simulink model "Smart_Grid_2"  (R2024b)
settings: Solver=FixedStepAuto  StartTime=0.0  StopTime=0.5  FixedStep=1e-5  RelTol=1e-3
undefined symbols (not defined in the file): Ion, Lithium
libraries: spsSeriesRLCBranchLib x76, spsRMSLib x65, spsIGBTDiodeLib x41, eeGeneralControl x36, slpidlib x34, spsThreePhaseVIMeasurementLib x32, spsVoltageMeasurementLib x18, simulink x16, spsCurrentMeasurementLib x15, spsThreePhaseBreakerLib x12, spsAlphaBetaZerotodq0Lib x12, spsPower3phPhasorLib x10
(part 3 of 8)

== system Smart_Grid_2/Battery_Farm, V2G 110KWH/Subsystem ==
  PWM1 : Inport
  PWM2 : Inport  Port=2
  PWM3 : Inport  Port=3
  PWM4 : Inport  Port=4
  PWM5 : Inport  Port=5
  PWM6 : Inport  Port=6
  IGBT/Diode{,1..5} (6 alike) : spsIGBTDiodeLib/IGBT//Diode  Ron=1e-3  Rs=1e5  Cs=inf  Measurements=off
  Series RLC Branch9 : spsSeriesRLCBranchLib/Series RLC Branch  LConnTagsString=__new0  RConnTagsString=__new0  BranchType=RC  Resistance=1e-3  Inductance=1e-3  SetiL0=off  InitialCurrent=0  Capacitance=5600e-6  Setx0=on  InitialVoltage=800  Measurements=None
  VR : PMIOPort  Side=Left
  VY : PMIOPort  Port=2  Side=Left
  VB : PMIOPort  Port=3  Side=Left
  VDC+ : PMIOPort  Port=4  Side=Right
  VDC- : PMIOPort  Port=5  Side=Right
  wires:
  PWM5/1 -> IGBT/Diode4/1
  PWM3/1 -> IGBT/Diode2/1
  PWM1/1 -> IGBT/Diode/1
  PWM2/1 -> IGBT/Diode1/1
  PWM6/1 -> IGBT/Diode5/1
  PWM4/1 -> IGBT/Diode3/1
  connections:
  IGBT/Diode1/RConn1 -- VDC-/RConn1 -- Series RLC Branch9/RConn1 -- IGBT/Diode5/RConn1 -- IGBT/Diode3/RConn1
  IGBT/Diode/RConn1 -- VR/RConn1 -- IGBT/Diode1/LConn1
  IGBT/Diode/LConn1 -- VDC+/RConn1 -- Series RLC Branch9/LConn1 -- IGBT/Diode4/LConn1 -- IGBT/Diode2/LConn1
  IGBT/Diode2/RConn1 -- VY/RConn1 -- IGBT/Diode3/LConn1
  IGBT/Diode4/RConn1 -- VB/RConn1 -- IGBT/Diode5/LConn1

== system Smart_Grid_2/Battery_Farm, V2G 110KWH/Subsystem1 ==
  Battery : spsBatteryLib/Battery  BatType=Lithium-Ion  NomV=360  NomQ=300  SOC=50  Batt_Tr=1  PresetModel=on  MaxQ=300  MinV=270  FullV=419.0354  Dis_rate=130.4348  R=0.012  Normal_OP=271.3043  expZone="[388.9389      14.73913]"
  Bus Selector : BusSelector  OutputSignals=SOC (%),Current (A),Voltage (V)
  + : PMIOPort  Side=Left
  - : PMIOPort  Port=2  Side=Left
  tag scope: Ibat=global, SOC=global, Vbat=global
  wires:
  Battery/1 -> Bus Selector/1
  Bus Selector/1 -> [SOC]  "<SOC (%)>"
  Bus Selector/2 -> [Ibat]  "<Current (A)>"
  Bus Selector/3 -> [Vbat]  "<Voltage (V)>"
  connections:
  Battery/LConn2 -- -/RConn1
  Battery/LConn1 -- +/RConn1

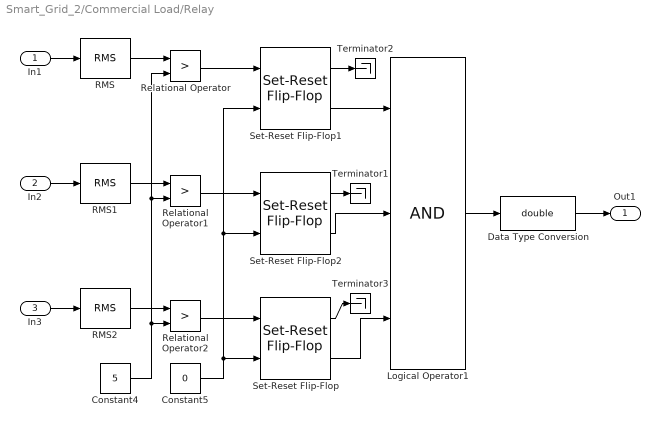
== system Smart_Grid_2/Commercial Load/Relay ==
  In1 : Inport
  In2 : Inport  Port=2
  In3 : Inport  Port=3
  Constant4 : Constant  Value=5
  Constant5 : Constant  Value=0
  Data Type Conversion : DataTypeConversion  OutDataTypeStr=double  SaturateOnIntegerOverflow=off  RndMeth=Floor
  Logical Operator1 : Logic  Inputs=3  AllPortsSameDT=off  OutDataTypeStr=boolean
  RMS : spsRMSLib/RMS  TrueRMS=on  Freq=50  RMSInit=0  Ts=0.001
  RMS1 : spsRMSLib/RMS  TrueRMS=on  Freq=50  RMSInit=0  Ts=0.001
  RMS2 : spsRMSLib/RMS  TrueRMS=on  Freq=50  RMSInit=0  Ts=0.001
  Relational Operator : RelationalOperator  Operator=>  OutDataTypeStr=boolean  RndMeth=Simplest  InputSameDT=off
  Relational Operator1 : RelationalOperator  Operator=>  OutDataTypeStr=boolean  RndMeth=Simplest  InputSameDT=off
  Relational Operator2 : RelationalOperator  Operator=>  OutDataTypeStr=boolean  RndMeth=Simplest  InputSameDT=off
  Set-Reset Flip-Flop : eeGeneralControl/Set-Reset Flip-Flop  LabelModeActiveChoice=Discrete  UndefState=Set  Q0=0  Ts=0.001
  Set-Reset Flip-Flop1 : eeGeneralControl/Set-Reset Flip-Flop  LabelModeActiveChoice=Discrete  UndefState=Set  Q0=0  Ts=0.001
  Set-Reset Flip-Flop2 : eeGeneralControl/Set-Reset Flip-Flop  LabelModeActiveChoice=Discrete  UndefState=Reset  Q0=0  Ts=0.001
  Terminator1 : Terminator
  Terminator2 : Terminator
  Terminator3 : Terminator
  Out1 : Outport
  wires:
  In2/1 -> RMS1/1
  Relational Operator1/1 -> Set-Reset Flip-Flop2/1
  Constant4/1 -> Relational Operator/2, Relational Operator1/2, Relational Operator2/2
  Constant5/1 -> Set-Reset Flip-Flop1/2, Set-Reset Flip-Flop2/2, Set-Reset Flip-Flop/2
  Logical Operator1/1 -> Data Type Conversion/1
  Data Type Conversion/1 -> Out1/1
  In3/1 -> RMS2/1
  In1/1 -> RMS/1
  RMS1/1 -> Relational Operator1/1
  RMS2/1 -> Relational Operator2/1
  RMS/1 -> Relational Operator/1
  Relational Operator2/1 -> Set-Reset Flip-Flop/1
  Relational Operator/1 -> Set-Reset Flip-Flop1/1
  Set-Reset Flip-Flop/2 -> Logical Operator1/3
  Set-Reset Flip-Flop2/2 -> Logical Operator1/2
  Set-Reset Flip-Flop1/2 -> Logical Operator1/1
  Set-Reset Flip-Flop2/1 -> Terminator1/1
  Set-Reset Flip-Flop/1 -> Terminator3/1
  Set-Reset Flip-Flop1/1 -> Terminator2/1

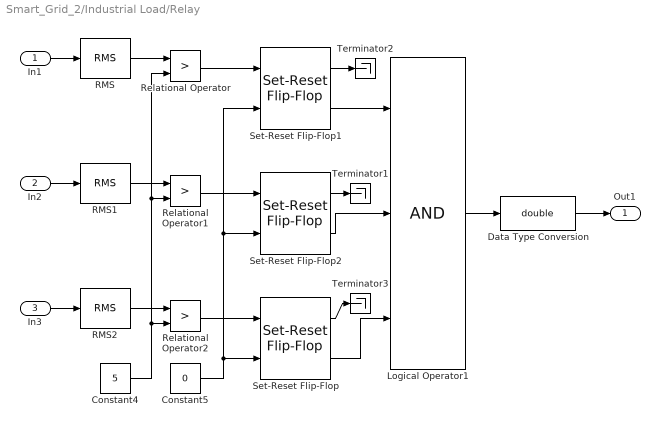
== system Smart_Grid_2/Industrial Load/Relay ==
  In1 : Inport
  In2 : Inport  Port=2
  In3 : Inport  Port=3
  Constant4 : Constant  Value=5
  Constant5 : Constant  Value=0
  Data Type Conversion : DataTypeConversion  OutDataTypeStr=double  SaturateOnIntegerOverflow=off  RndMeth=Floor
  Logical Operator1 : Logic  Inputs=3  AllPortsSameDT=off  OutDataTypeStr=boolean
  RMS : spsRMSLib/RMS  TrueRMS=on  Freq=50  RMSInit=0  Ts=0.001
  RMS1 : spsRMSLib/RMS  TrueRMS=on  Freq=50  RMSInit=0  Ts=0.001
  RMS2 : spsRMSLib/RMS  TrueRMS=on  Freq=50  RMSInit=0  Ts=0.001
  Relational Operator : RelationalOperator  Operator=>  OutDataTypeStr=boolean  RndMeth=Simplest  InputSameDT=off
  Relational Operator1 : RelationalOperator  Operator=>  OutDataTypeStr=boolean  RndMeth=Simplest  InputSameDT=off
  Relational Operator2 : RelationalOperator  Operator=>  OutDataTypeStr=boolean  RndMeth=Simplest  InputSameDT=off
  Set-Reset Flip-Flop : eeGeneralControl/Set-Reset Flip-Flop  LabelModeActiveChoice=Discrete  UndefState=Set  Q0=0  Ts=0.001
  Set-Reset Flip-Flop1 : eeGeneralControl/Set-Reset Flip-Flop  LabelModeActiveChoice=Discrete  UndefState=Set  Q0=0  Ts=0.001
  Set-Reset Flip-Flop2 : eeGeneralControl/Set-Reset Flip-Flop  LabelModeActiveChoice=Discrete  UndefState=Reset  Q0=0  Ts=0.001
  Terminator1 : Terminator
  Terminator2 : Terminator
  Terminator3 : Terminator
  Out1 : Outport
  wires:
  In2/1 -> RMS1/1
  Relational Operator1/1 -> Set-Reset Flip-Flop2/1
  Constant4/1 -> Relational Operator/2, Relational Operator1/2, Relational Operator2/2
  Constant5/1 -> Set-Reset Flip-Flop1/2, Set-Reset Flip-Flop2/2, Set-Reset Flip-Flop/2
  Logical Operator1/1 -> Data Type Conversion/1
  Data Type Conversion/1 -> Out1/1
  In3/1 -> RMS2/1
  In1/1 -> RMS/1
  RMS1/1 -> Relational Operator1/1
  RMS2/1 -> Relational Operator2/1
  RMS/1 -> Relational Operator/1
  Relational Operator2/1 -> Set-Reset Flip-Flop/1
  Relational Operator/1 -> Set-Reset Flip-Flop1/1
  Set-Reset Flip-Flop/2 -> Logical Operator1/3
  Set-Reset Flip-Flop2/2 -> Logical Operator1/2
  Set-Reset Flip-Flop1/2 -> Logical Operator1/1
  Set-Reset Flip-Flop2/1 -> Terminator1/1
  Set-Reset Flip-Flop/1 -> Terminator3/1
  Set-Reset Flip-Flop1/1 -> Terminator2/1

== system Smart_Grid_2/Residential Load 1/Relay ==
  In1 : Inport
  In2 : Inport  Port=2
  In3 : Inport  Port=3
  Constant4 : Constant  Value=5
  Constant5 : Constant  Value=0
  Data Type Conversion : DataTypeConversion  OutDataTypeStr=double  SaturateOnIntegerOverflow=off  RndMeth=Floor
  Logical Operator1 : Logic  Inputs=3  AllPortsSameDT=off  OutDataTypeStr=boolean
  RMS : spsRMSLib/RMS  TrueRMS=on  Freq=50  RMSInit=0  Ts=0.001
  RMS1 : spsRMSLib/RMS  TrueRMS=on  Freq=50  RMSInit=0  Ts=0.001
  RMS2 : spsRMSLib/RMS  TrueRMS=on  Freq=50  RMSInit=0  Ts=0.001
  Relational Operator : RelationalOperator  Operator=>  OutDataTypeStr=boolean  RndMeth=Simplest  InputSameDT=off
  Relational Operator1 : RelationalOperator  Operator=>  OutDataTypeStr=boolean  RndMeth=Simplest  InputSameDT=off
  Relational Operator2 : RelationalOperator  Operator=>  OutDataTypeStr=boolean  RndMeth=Simplest  InputSameDT=off
  Set-Reset Flip-Flop : eeGeneralControl/Set-Reset Flip-Flop  LabelModeActiveChoice=Discrete  UndefState=Set  Q0=0  Ts=0.001
  Set-Reset Flip-Flop1 : eeGeneralControl/Set-Reset Flip-Flop  LabelModeActiveChoice=Discrete  UndefState=Set  Q0=0  Ts=0.001
  Set-Reset Flip-Flop2 : eeGeneralControl/Set-Reset Flip-Flop  LabelModeActiveChoice=Discrete  UndefState=Reset  Q0=0  Ts=0.001
  Terminator1 : Terminator
  Terminator2 : Terminator
  Terminator3 : Terminator
  Out1 : Outport
  wires:
  In2/1 -> RMS1/1
  Relational Operator1/1 -> Set-Reset Flip-Flop2/1
  Constant4/1 -> Relational Operator/2, Relational Operator1/2, Relational Operator2/2
  Constant5/1 -> Set-Reset Flip-Flop1/2, Set-Reset Flip-Flop2/2, Set-Reset Flip-Flop/2
  Logical Operator1/1 -> Data Type Conversion/1
  Data Type Conversion/1 -> Out1/1
  In3/1 -> RMS2/1
  In1/1 -> RMS/1
  RMS1/1 -> Relational Operator1/1
  RMS2/1 -> Relational Operator2/1
  RMS/1 -> Relational Operator/1
  Relational Operator2/1 -> Set-Reset Flip-Flop/1
  Relational Operator/1 -> Set-Reset Flip-Flop1/1
  Set-Reset Flip-Flop/2 -> Logical Operator1/3
  Set-Reset Flip-Flop2/2 -> Logical Operator1/2
  Set-Reset Flip-Flop1/2 -> Logical Operator1/1
  Set-Reset Flip-Flop2/1 -> Terminator1/1
  Set-Reset Flip-Flop/1 -> Terminator3/1
  Set-Reset Flip-Flop1/1 -> Terminator2/1

== system Smart_Grid_2/Residential Load 2/Relay ==
  In1 : Inport
  In2 : Inport  Port=2
  In3 : Inport  Port=3
  Constant4 : Constant  Value=5
  Constant5 : Constant  Value=0
  Data Type Conversion : DataTypeConversion  OutDataTypeStr=double  SaturateOnIntegerOverflow=off  RndMeth=Floor
  Logical Operator1 : Logic  Inputs=3  AllPortsSameDT=off  OutDataTypeStr=boolean
  RMS : spsRMSLib/RMS  TrueRMS=on  Freq=50  RMSInit=0  Ts=0.001
  RMS1 : spsRMSLib/RMS  TrueRMS=on  Freq=50  RMSInit=0  Ts=0.001
  RMS2 : spsRMSLib/RMS  TrueRMS=on  Freq=50  RMSInit=0  Ts=0.001
  Relational Operator : RelationalOperator  Operator=>  OutDataTypeStr=boolean  RndMeth=Simplest  InputSameDT=off
  Relational Operator1 : RelationalOperator  Operator=>  OutDataTypeStr=boolean  RndMeth=Simplest  InputSameDT=off
  Relational Operator2 : RelationalOperator  Operator=>  OutDataTypeStr=boolean  RndMeth=Simplest  InputSameDT=off
  Set-Reset Flip-Flop : eeGeneralControl/Set-Reset Flip-Flop  LabelModeActiveChoice=Discrete  UndefState=Set  Q0=0  Ts=0.001
  Set-Reset Flip-Flop1 : eeGeneralControl/Set-Reset Flip-Flop  LabelModeActiveChoice=Discrete  UndefState=Set  Q0=0  Ts=0.001
  Set-Reset Flip-Flop2 : eeGeneralControl/Set-Reset Flip-Flop  LabelModeActiveChoice=Discrete  UndefState=Reset  Q0=0  Ts=0.001
  Terminator1 : Terminator
  Terminator2 : Terminator
  Terminator3 : Terminator
  Out1 : Outport
  wires:
  In2/1 -> RMS1/1
  Relational Operator1/1 -> Set-Reset Flip-Flop2/1
  Constant4/1 -> Relational Operator/2, Relational Operator1/2, Relational Operator2/2
  Constant5/1 -> Set-Reset Flip-Flop1/2, Set-Reset Flip-Flop2/2, Set-Reset Flip-Flop/2
  Logical Operator1/1 -> Data Type Conversion/1
  Data Type Conversion/1 -> Out1/1
  In3/1 -> RMS2/1
  In1/1 -> RMS/1
  RMS1/1 -> Relational Operator1/1
  RMS2/1 -> Relational Operator2/1
  RMS/1 -> Relational Operator/1
  Relational Operator2/1 -> Set-Reset Flip-Flop/1
  Relational Operator/1 -> Set-Reset Flip-Flop1/1
  Set-Reset Flip-Flop/2 -> Logical Operator1/3
  Set-Reset Flip-Flop2/2 -> Logical Operator1/2
  Set-Reset Flip-Flop1/2 -> Logical Operator1/1
  Set-Reset Flip-Flop2/1 -> Terminator1/1
  Set-Reset Flip-Flop/1 -> Terminator3/1
  Set-Reset Flip-Flop1/1 -> Terminator2/1

== system Smart_Grid_2/Residential Load 3/Relay ==
  In1 : Inport
  In2 : Inport  Port=2
  In3 : Inport  Port=3
  Constant4 : Constant  Value=5
  Constant5 : Constant  Value=0
  Data Type Conversion : DataTypeConversion  OutDataTypeStr=double  SaturateOnIntegerOverflow=off  RndMeth=Floor
  Logical Operator1 : Logic  Inputs=3  AllPortsSameDT=off  OutDataTypeStr=boolean
  RMS : spsRMSLib/RMS  TrueRMS=on  Freq=50  RMSInit=0  Ts=0.001
  RMS1 : spsRMSLib/RMS  TrueRMS=on  Freq=50  RMSInit=0  Ts=0.001
  RMS2 : spsRMSLib/RMS  TrueRMS=on  Freq=50  RMSInit=0  Ts=0.001
  Relational Operator : RelationalOperator  Operator=>  OutDataTypeStr=boolean  RndMeth=Simplest  InputSameDT=off
  Relational Operator1 : RelationalOperator  Operator=>  OutDataTypeStr=boolean  RndMeth=Simplest  InputSameDT=off
  Relational Operator2 : RelationalOperator  Operator=>  OutDataTypeStr=boolean  RndMeth=Simplest  InputSameDT=off
  Set-Reset Flip-Flop : eeGeneralControl/Set-Reset Flip-Flop  LabelModeActiveChoice=Discrete  UndefState=Set  Q0=0  Ts=0.001
  Set-Reset Flip-Flop1 : eeGeneralControl/Set-Reset Flip-Flop  LabelModeActiveChoice=Discrete  UndefState=Set  Q0=0  Ts=0.001
  Set-Reset Flip-Flop2 : eeGeneralControl/Set-Reset Flip-Flop  LabelModeActiveChoice=Discrete  UndefState=Reset  Q0=0  Ts=0.001
  Terminator1 : Terminator
  Terminator2 : Terminator
  Terminator3 : Terminator
  Out1 : Outport
  wires:
  In2/1 -> RMS1/1
  Relational Operator1/1 -> Set-Reset Flip-Flop2/1
  Constant4/1 -> Relational Operator/2, Relational Operator1/2, Relational Operator2/2
  Constant5/1 -> Set-Reset Flip-Flop1/2, Set-Reset Flip-Flop2/2, Set-Reset Flip-Flop/2
  Logical Operator1/1 -> Data Type Conversion/1
  Data Type Conversion/1 -> Out1/1
  In3/1 -> RMS2/1
  In1/1 -> RMS/1
  RMS1/1 -> Relational Operator1/1
  RMS2/1 -> Relational Operator2/1
  RMS/1 -> Relational Operator/1
  Relational Operator2/1 -> Set-Reset Flip-Flop/1
  Relational Operator/1 -> Set-Reset Flip-Flop1/1
  Set-Reset Flip-Flop/2 -> Logical Operator1/3
  Set-Reset Flip-Flop2/2 -> Logical Operator1/2
  Set-Reset Flip-Flop1/2 -> Logical Operator1/1
  Set-Reset Flip-Flop2/1 -> Terminator1/1
  Set-Reset Flip-Flop/1 -> Terminator3/1
  Set-Reset Flip-Flop1/1 -> Terminator2/1

== system Smart_Grid_2/Solar_Farm 100KW/Relay ==
  In1 : Inport
  In2 : Inport  Port=2
  In3 : Inport  Port=3
  Constant4 : Constant  Value=7
  Constant5 : Constant  Value=0
  Data Type Conversion : DataTypeConversion  OutDataTypeStr=double  SaturateOnIntegerOverflow=off  RndMeth=Floor
  Logical Operator1 : Logic  Inputs=3  AllPortsSameDT=off  OutDataTypeStr=boolean
  RMS : spsRMSLib/RMS  TrueRMS=on  Freq=50  RMSInit=0  Ts=0.001
  RMS1 : spsRMSLib/RMS  TrueRMS=on  Freq=50  RMSInit=0  Ts=0.001
  RMS2 : spsRMSLib/RMS  TrueRMS=on  Freq=50  RMSInit=0  Ts=0.001
  Relational Operator : RelationalOperator  Operator=>  OutDataTypeStr=boolean  RndMeth=Simplest  InputSameDT=off
  Relational Operator1 : RelationalOperator  Operator=>  OutDataTypeStr=boolean  RndMeth=Simplest  InputSameDT=off
  Relational Operator2 : RelationalOperator  Operator=>  OutDataTypeStr=boolean  RndMeth=Simplest  InputSameDT=off
  Set-Reset Flip-Flop : eeGeneralControl/Set-Reset Flip-Flop  LabelModeActiveChoice=Discrete  UndefState=Set  Q0=0  Ts=0.001
  Set-Reset Flip-Flop1 : eeGeneralControl/Set-Reset Flip-Flop  LabelModeActiveChoice=Discrete  UndefState=Set  Q0=0  Ts=0.001
  Set-Reset Flip-Flop2 : eeGeneralControl/Set-Reset Flip-Flop  LabelModeActiveChoice=Discrete  UndefState=Reset  Q0=0  Ts=0.001
  Terminator1 : Terminator
  Terminator2 : Terminator
  Terminator3 : Terminator
  Out1 : Outport
  wires:
  In2/1 -> RMS1/1
  Relational Operator1/1 -> Set-Reset Flip-Flop2/1
  Constant4/1 -> Relational Operator/2, Relational Operator1/2, Relational Operator2/2
  Constant5/1 -> Set-Reset Flip-Flop1/2, Set-Reset Flip-Flop2/2, Set-Reset Flip-Flop/2
  Logical Operator1/1 -> Data Type Conversion/1
  Data Type Conversion/1 -> Out1/1
  In3/1 -> RMS2/1
  In1/1 -> RMS/1
  RMS1/1 -> Relational Operator1/1
  RMS2/1 -> Relational Operator2/1
  RMS/1 -> Relational Operator/1
  Relational Operator2/1 -> Set-Reset Flip-Flop/1
  Relational Operator/1 -> Set-Reset Flip-Flop1/1
  Set-Reset Flip-Flop/2 -> Logical Operator1/3
  Set-Reset Flip-Flop2/2 -> Logical Operator1/2
  Set-Reset Flip-Flop1/2 -> Logical Operator1/1
  Set-Reset Flip-Flop2/1 -> Terminator1/1
  Set-Reset Flip-Flop/1 -> Terminator3/1
  Set-Reset Flip-Flop1/1 -> Terminator2/1
